simulink model "compare_convertions"  (R2023b)
settings: Solver=VariableStepAuto  StartTime=0.0  StopTime=t(end)  RelTol=1e-3
settings Model: Creator=franc  LastModifiedBy=franc

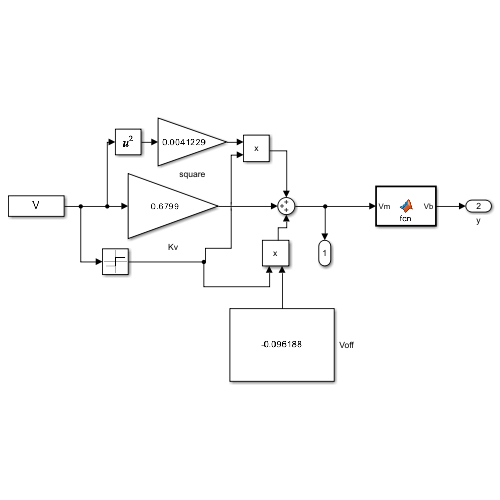
[thumbnail: Simulink's stored preview of the top-level diagram]
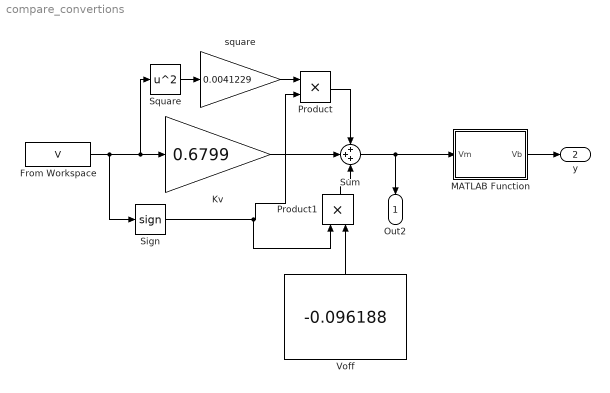
== system compare_convertions ==
  From Workspace : FromWorkspace  VariableName=V  SampleTime=t(2)-t(1)
  Kv : Gain  Gain=0.6799
  MATLAB Function : MATLAB Function  TreatAsAtomicUnit=on
  Product : Product
  Product1 : Product
  Sign : Signum
  Square : Math  Operator=square
  Sum : Sum  Inputs=+++
  Voff : Constant  Value=-0.096188
  square : Gain  Gain=0.0041229
  Out2 : Outport
  y : Outport  Port=2
  wires:
  square/1 -> Product/1
  From Workspace/1 -> Sign/1, Square/1, Kv/1
  Voff/1 -> Product1/2
  Sign/1 -> Product1/1, Product/2
  Product1/1 -> Sum/3
  Product/1 -> Sum/1
  Kv/1 -> Sum/2
  Square/1 -> square/1
  Sum/1 -> Out2/1, MATLAB Function/1(Vm)
  MATLAB Function/1(Vb) -> y/1

== matlab function compare_convertions/MATLAB Function ==
  data: Vm input; Vb output
function Vb = fcn(Vm)
Vb=Vm2Vb(Vm);
end
